simulink model "week1problem2"  (R2020a)
settings: Solver=VariableStepAuto  StartTime=0.0  StopTime=10.0  RelTol=1e-3
values from neighbouring files (symbols this model uses):
  B = 1000    [week1problem2.mat]
  K1 = 36000    [week1problem2.mat]
  K2 = 204034    [week1problem2.mat]
  M1 = 600    [week1problem2.mat]
  M2 = 90    [week1problem2.mat]
settings Model: Creator=Admin  LastModifiedBy=Admin

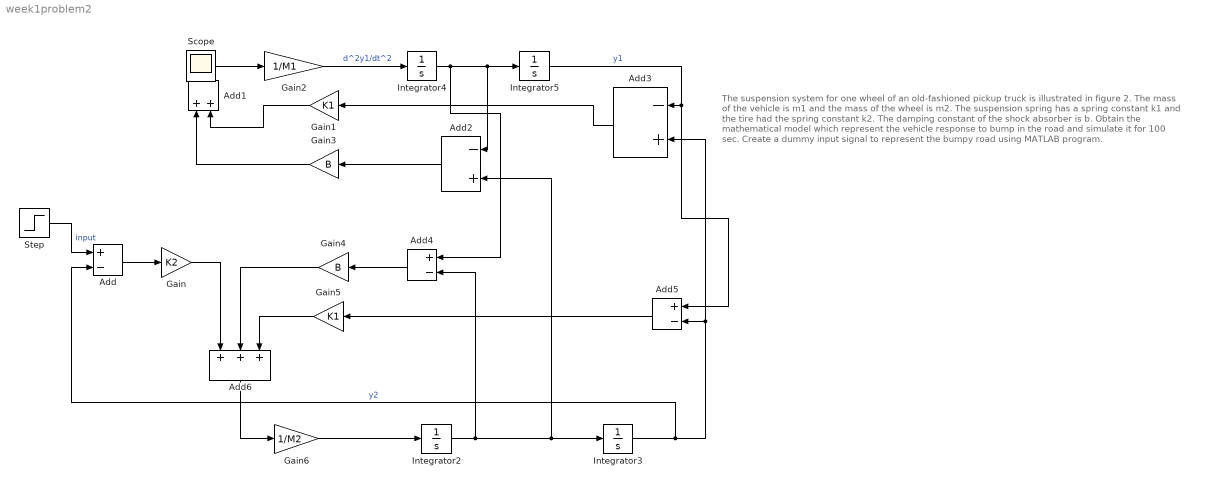
== system week1problem2 ==
  note: The suspension system for one wheel of an old-fashioned pickup truck is illustrated in figure 2. The mass of the vehicle is m1 and the mass of the wheel is m2. The suspension spring has a spring constant k1 and the tire had the spring constant k2. The damping constant of the shock absorber is b. Obtain the mathematical model which represent the vehicle response to bump in the road and simulate it for 100 sec. Create a dummy input signal to represent the bumpy road using MATLAB program.
  Add : Sum  Inputs=+-
  Add1 : Sum
  Add2 : Sum  Inputs=-+
  Add3 : Sum  Inputs=-+
  Add4 : Sum  Inputs=+-
  Add5 : Sum  Inputs=+-
  Add6 : Sum  Inputs=+++
  Gain : Gain  Gain=K2
  Gain1 : Gain  Gain=K1
  Gain2 : Gain  Gain=1/M1
  Gain3 : Gain  Gain=B
  Gain4 : Gain  Gain=B
  Gain5 : Gain  Gain=K1
  Gain6 : Gain  Gain=1/M2
  Integrator{2..5} (4 alike) : Integrator
  Step : Step  SampleTime=0
  Scope : Scope
  wires:
  Gain1/1 -> Add1/2
  Integrator3/1 -> Add/2, Add5/2, Add3/2  "y2"
  Gain2/1 -> Integrator4/1  "d^2y1/dt^2"
  Integrator5/1 -> Add5/1, Add3/1  "y1"
  Add3/1 -> Gain1/1
  Gain4/1 -> Add6/2
  Integrator2/1 -> Add4/2, Add2/2, Integrator3/1
  Add5/1 -> Gain5/1
  Add4/1 -> Gain4/1
  Add2/1 -> Gain3/1
  Add6/1 -> Gain6/1
  Gain5/1 -> Add6/3
  Add/1 -> Gain/1
  Step/1 -> Add/1  "input"
  Add1/1 -> Gain2/1
  Gain6/1 -> Integrator2/1
  Gain3/1 -> Add1/1
  Integrator4/1 -> Add4/1, Add2/1, Integrator5/1
  Gain/1 -> Add6/1
